simulink model "que5"  (R2020b)
settings: Solver=VariableStepAuto  StartTime=0.0  StopTime=10.0  RelTol=1e-3
settings Model: Creator=ANUJA  LastModifiedBy=ANUJA

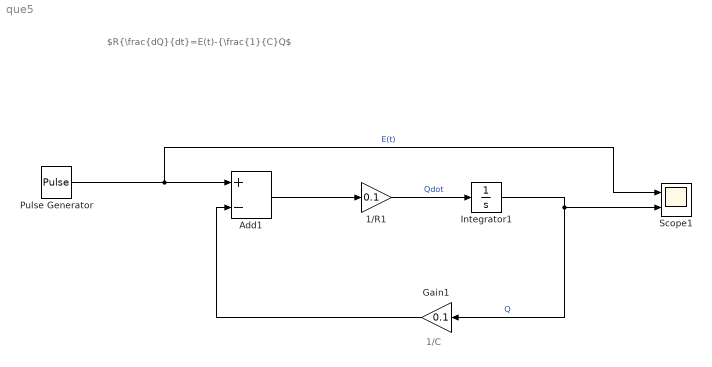
== system que5 ==
  note: $R{\frac{dQ}{dt}=E(t)-{\frac{1}{C}Q$
  note: 1/C
  1/R1 : Gain  Gain=0.1
  Add1 : Sum  Inputs=+-
  Gain1 : Gain  Gain=0.1
  Integrator1 : Integrator  InitialCondition=5
  Pulse Generator : DiscretePulseGenerator  Amplitude=5
  Scope1 : Scope  NumInputPorts=2
  wires:
  Gain1/1 -> Add1/2
  1/R1/1 -> Integrator1/1  "Qdot"
  Add1/1 -> 1/R1/1
  Integrator1/1 -> Gain1/1, Scope1/2  "Q"
  Pulse Generator/1 -> Scope1/1, Add1/1  "E(t)"
